simulink model "chap9_5sim"  (Simulink 5.0)
settings: Solver=ode45  StartTime=0.0  StopTime=30  FixedStep=0.001  RelTol=1e-3
settings Model: LastModifiedBy=Administrator  ExtModeTrigMode=oneshot  ExtModeArmWhenConnect=off  LimitDataPoints=off  BooleanDataType=off

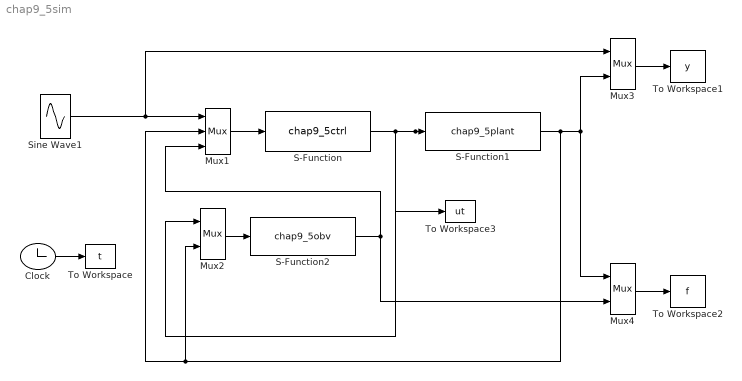
== system chap9_5sim ==
  Clock : Clock
  Mux1 : Mux  Inputs=3
  Mux2 : Mux  Inputs=2
  Mux3 : Mux  Inputs=2
  Mux4 : Mux  Inputs=2
  S-Function : S-Function  FunctionName=chap9_5ctrl
  S-Function1 : S-Function  FunctionName=chap9_5plant
  S-Function2 : S-Function  FunctionName=chap9_5obv
  Sine Wave1 : Sin  SampleTime=0
  To Workspace : ToWorkspace  VariableName=t  SampleTime=-1  SaveFormat=Array
  To Workspace1 : ToWorkspace  VariableName=y  SampleTime=-1  SaveFormat=Array
  To Workspace2 : ToWorkspace  VariableName=f  SampleTime=-1  SaveFormat=Array
  To Workspace3 : ToWorkspace  VariableName=ut  SampleTime=-1  SaveFormat=Array
  wires:
  Mux3/1 -> To Workspace1/1
  S-Function/1 -> S-Function1/1, Mux2/1, To Workspace3/1
  Sine Wave1/1 -> Mux1/1, Mux3/1
  S-Function1/1 -> Mux1/2, Mux2/2, Mux3/2, Mux4/1
  Clock/1 -> To Workspace/1
  Mux1/1 -> S-Function/1
  Mux2/1 -> S-Function2/1
  S-Function2/1 -> Mux1/3, Mux4/2
  Mux4/1 -> To Workspace2/1
